simulink model "FIR"  (R2018a)
settings: Solver=VariableStepAuto  StartTime=0.0  StopTime=0.005  RelTol=1e-3
libraries: xbsIndex_r4 x51
settings Model: Creator=57315  LastModifiedBy=57315

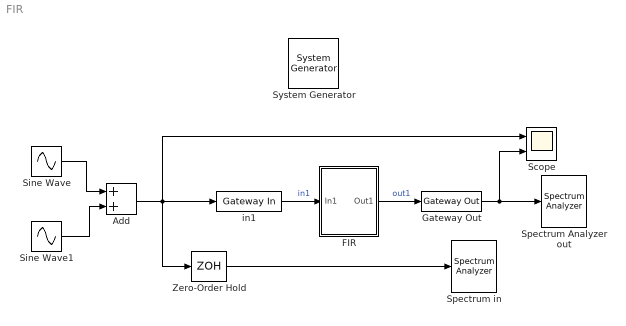
== system FIR ==
  " System Generator" : xbsIndex_r4/ System Generator  Tag=genX  xilinxfamily=kintex7  part=xc7k325t  speed=-3  package=fbg676  synthesis_tool=Vivado  clock_wrapper=Clock Enables  directory=G:/a_max/max_xilinx/max/System_Generator/FIR/FIR3/par  proj_type=Vivado  Synth_file=Vivado Synthesis Defaults  Impl_file=Vivado Implementation Defaults  testbench=on  simulink_period=1/50e6  sysclk_period=20  dcm_input_clock_period=10  incr_netlist=off  trim_vbits=Everywhere in SubSystem  dbl_ovrd=According to Block Masks  core_generation=According to Block Masks  run_coregen=off  deprecated_control=off  eval_field=0  block_type=sysgen
  Add : Sum
  "FIR " : Subsystem
  Gateway Out : xbsIndex_r4/Gateway Out  inherit_from_input=off  hdl_port=on  rows=1  columns=1  UseAsDAC=off  DACChannel='1'  interface=None  automatic_assignment=on  address_offset=hex2dec('00')  intf_name=''  intf_description=''  timing_constraint=None  locs_specified=off  LOCs={}  io_standard={}  block_type=gatewayout
  Scope : Scope  NumInputPorts=2
  Sine Wave : Sin  Frequency=2*pi*1e6  SampleTime=0
  Sine Wave1 : Sin  Frequency=2*pi*9e6  SampleTime=0
  Spectrum Analyzer out : SpectrumAnalyzer
  Spectrum in : SpectrumAnalyzer
  Zero-Order Hold : ZeroOrderHold  SampleTime=1/50e6
  in1 : xbsIndex_r4/Gateway In  gui_display_data_type=Fixed-point  arith_type="Signed  (2's comp)"  n_bits=16  bin_pt=14  preci_type=Single  exp_width=8  frac_width=24  rows=1  columns=1  quantization="Round  (unbiased: +/- Inf)"  overflow=Saturate  period=1/50e6  UseAsADC=off  ADCChannel='1'  interface=None  automatic_assignment=on  address_offset=hex2dec('00')  intf_name=''  intf_description=''  default_value=0  timing_constraint=None  locs_specified=off  LOCs={}  io_standard={}  inherit_from_input=off  hdl_port=on  dbl_ovrd=off  block_type=gatewayin
  wires:
  in1/1 -> "FIR "/1(In1)  "in1"
  Sine Wave/1 -> Add/1
  Sine Wave1/1 -> Add/2
  Add/1 -> Scope/1, Zero-Order Hold/1, in1/1
  Gateway Out/1 -> Scope/2, Spectrum Analyzer out/1
  Zero-Order Hold/1 -> Spectrum in/1
  "FIR "/1(Out1) -> Gateway Out/1  "out1"

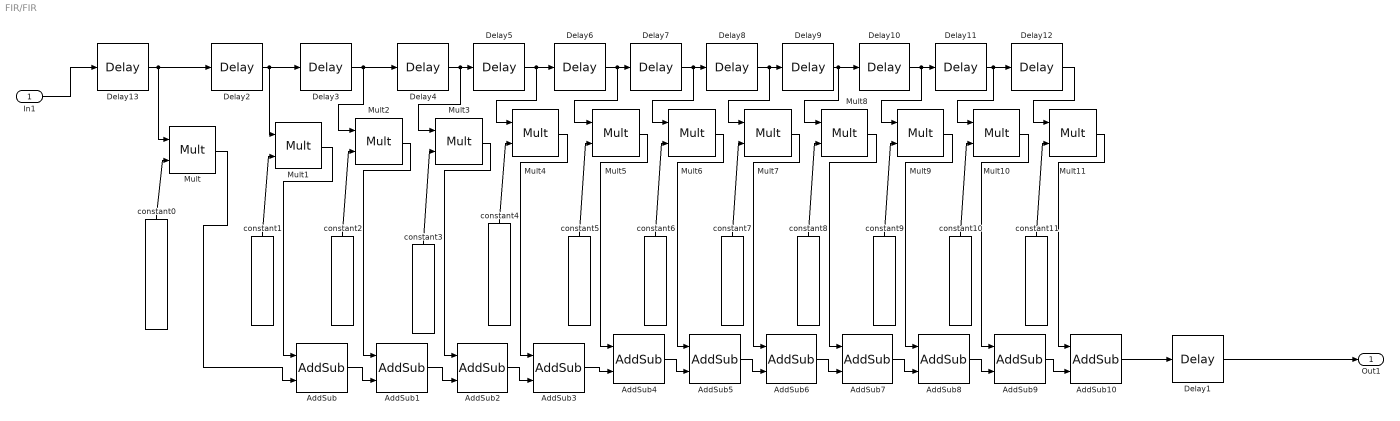
== system FIR/FIR  ==
  In1 : Inport
  AddSub : xbsIndex_r4/AddSub  mode=Addition  use_carryin=off  use_carryout=off  en=off  latency=0  precision=Full  arith_type=Unsigned  n_bits=16  bin_pt=14  quantization=Truncate  overflow=Wrap  use_behavioral_HDL=off  hw_selection=Fabric  pipelined=off  dbl_ovrd=off  block_type=addsub
  AddSub{1..10} (10 alike) : xbsIndex_r4/AddSub  mode=Addition  use_carryin=off  use_carryout=off  en=off  latency=1  precision=Full  arith_type=Unsigned  n_bits=16  bin_pt=14  quantization=Truncate  overflow=Wrap  use_behavioral_HDL=off  hw_selection=Fabric  pipelined=off  dbl_ovrd=off  block_type=addsub
  Delay1 : xbsIndex_r4/Delay  rst=off  infoeditControl=Selection of Reset will increase slice count due to use of real FFs and instead of SRLs  en=off  latency=1  reg_retiming=off  dbl_ovrd=off  block_type=delay
  Delay{2..12} (11 alike) : xbsIndex_r4/Delay  rst=off  infoeditControl=Selection of Reset will increase slice count due to use of real FFs and instead of SRLs  en=off  latency=2  reg_retiming=off  dbl_ovrd=off  block_type=delay
  Delay13 : xbsIndex_r4/Delay  rst=off  infoeditControl=Selection of Reset will increase slice count due to use of real FFs and instead of SRLs  en=off  latency=1  reg_retiming=off  dbl_ovrd=off  block_type=delay
  Mult{,1..11} (12 alike) : xbsIndex_r4/Mult  precision=Full  arith_type="Signed  (2's comp)"  n_bits=16  bin_pt=14  quantization=Truncate  overflow=Wrap  en=off  latency=3  use_behavioral_HDL=off  opt=Speed  use_embedded=on  optimum_pipeline=off  pipeline=on  dbl_ovrd=off  use_rpm=on  placement_style=Triangular  block_type=mult
  constant0 : xbsIndex_r4/Constant  const=1.242e-02  gui_display_data_type=Fixed-point  arith_type=Signed (2's comp)  n_bits=16  bin_pt=14  preci_type=Single  exp_width=8  frac_width=24  explicit_period=off  period=1  equ=P=C  opselect=C  inp2=PCIN>>17  opr=+  inp1=P  carry=CIN  dbl_ovrd=off  block_type=constant
  constant1 : xbsIndex_r4/Constant  const=2.442e-02  gui_display_data_type=Fixed-point  arith_type=Signed (2's comp)  n_bits=16  bin_pt=14  preci_type=Single  exp_width=8  frac_width=24  explicit_period=off  period=1  equ=P=C  opselect=C  inp2=PCIN>>17  opr=+  inp1=P  carry=CIN  dbl_ovrd=off  block_type=constant
  constant10 : xbsIndex_r4/Constant  const=2.442e-02  gui_display_data_type=Fixed-point  arith_type=Signed (2's comp)  n_bits=16  bin_pt=14  preci_type=Single  exp_width=8  frac_width=24  explicit_period=off  period=1  equ=P=C  opselect=C  inp2=PCIN>>17  opr=+  inp1=P  carry=CIN  dbl_ovrd=off  block_type=constant
  constant11 : xbsIndex_r4/Constant  const=1.242e-02  gui_display_data_type=Fixed-point  arith_type=Signed (2's comp)  n_bits=16  bin_pt=14  preci_type=Single  exp_width=8  frac_width=24  explicit_period=off  period=1  equ=P=C  opselect=C  inp2=PCIN>>17  opr=+  inp1=P  carry=CIN  dbl_ovrd=off  block_type=constant
  constant2 : xbsIndex_r4/Constant  const=5.688e-02  gui_display_data_type=Fixed-point  arith_type=Signed (2's comp)  n_bits=16  bin_pt=14  preci_type=Single  exp_width=8  frac_width=24  explicit_period=off  period=1  equ=P=C  opselect=C  inp2=PCIN>>17  opr=+  inp1=P  carry=CIN  dbl_ovrd=off  block_type=constant
  constant3 : xbsIndex_r4/Constant  const=.1003  gui_display_data_type=Fixed-point  arith_type=Signed (2's comp)  n_bits=16  bin_pt=14  preci_type=Single  exp_width=8  frac_width=24  explicit_period=off  period=1  equ=P=C  opselect=C  inp2=PCIN>>17  opr=+  inp1=P  carry=CIN  dbl_ovrd=off  block_type=constant
  constant4 : xbsIndex_r4/Constant  const=0.1408  gui_display_data_type=Fixed-point  arith_type=Signed (2's comp)  n_bits=16  bin_pt=14  preci_type=Single  exp_width=8  frac_width=24  explicit_period=off  period=1  equ=P=C  opselect=C  inp2=PCIN>>17  opr=+  inp1=P  carry=CIN  dbl_ovrd=off  block_type=constant
  constant5 : xbsIndex_r4/Constant  const=.1652  gui_display_data_type=Fixed-point  arith_type=Signed (2's comp)  n_bits=16  bin_pt=14  preci_type=Single  exp_width=8  frac_width=24  explicit_period=off  period=1  equ=P=C  opselect=C  inp2=PCIN>>17  opr=+  inp1=P  carry=CIN  dbl_ovrd=off  block_type=constant
  constant6 : xbsIndex_r4/Constant  const=.1625  gui_display_data_type=Fixed-point  arith_type=Signed (2's comp)  n_bits=16  bin_pt=14  preci_type=Single  exp_width=8  frac_width=24  explicit_period=off  period=1  equ=P=C  opselect=C  inp2=PCIN>>17  opr=+  inp1=P  carry=CIN  dbl_ovrd=off  block_type=constant
  constant7 : xbsIndex_r4/Constant  const=.1408  gui_display_data_type=Fixed-point  arith_type=Signed (2's comp)  n_bits=16  bin_pt=14  preci_type=Single  exp_width=8  frac_width=24  explicit_period=off  period=1  equ=P=C  opselect=C  inp2=PCIN>>17  opr=+  inp1=P  carry=CIN  dbl_ovrd=off  block_type=constant
  constant8 : xbsIndex_r4/Constant  const=.1003  gui_display_data_type=Fixed-point  arith_type=Signed (2's comp)  n_bits=16  bin_pt=14  preci_type=Single  exp_width=8  frac_width=24  explicit_period=off  period=1  equ=P=C  opselect=C  inp2=PCIN>>17  opr=+  inp1=P  carry=CIN  dbl_ovrd=off  block_type=constant
  constant9 : xbsIndex_r4/Constant  const=5.688e-02  gui_display_data_type=Fixed-point  arith_type=Signed (2's comp)  n_bits=16  bin_pt=14  preci_type=Single  exp_width=8  frac_width=24  explicit_period=off  period=1  equ=P=C  opselect=C  inp2=PCIN>>17  opr=+  inp1=P  carry=CIN  dbl_ovrd=off  block_type=constant
  Out1 : Outport
  wires:
  AddSub2/1 -> AddSub3/2
  Mult6/1 -> AddSub5/1
  Delay4/1 -> Delay5/1, Mult3/1
  In1/1 -> Delay13/1
  AddSub/1 -> AddSub1/2
  AddSub3/1 -> AddSub4/2
  constant1/1 -> Mult1/2
  Delay2/1 -> Delay3/1, Mult1/1
  Mult10/1 -> AddSub9/1
  constant6/1 -> Mult6/2
  Mult3/1 -> AddSub2/1
  Mult2/1 -> AddSub1/1
  constant2/1 -> Mult2/2
  Delay13/1 -> Mult/1, Delay2/1
  Mult1/1 -> AddSub/1
  Delay6/1 -> Delay7/1, Mult5/1
  constant3/1 -> Mult3/2
  AddSub9/1 -> AddSub10/2
  Mult11/1 -> AddSub10/1
  Mult/1 -> AddSub/2
  constant9/1 -> Mult9/2
  Delay1/1 -> Out1/1
  constant7/1 -> Mult7/2
  constant0/1 -> Mult/2
  constant8/1 -> Mult8/2
  AddSub6/1 -> AddSub7/2
  AddSub1/1 -> AddSub2/2
  constant4/1 -> Mult4/2
  Delay12/1 -> Mult11/1
  AddSub10/1 -> Delay1/1
  AddSub7/1 -> AddSub8/2
  Delay9/1 -> Mult8/1, Delay10/1
  constant11/1 -> Mult11/2
  Delay8/1 -> Delay9/1, Mult7/1
  Mult5/1 -> AddSub4/1
  Delay11/1 -> Mult10/1, Delay12/1
  Mult7/1 -> AddSub6/1
  constant10/1 -> Mult10/2
  Delay3/1 -> Delay4/1, Mult2/1
  Delay7/1 -> Delay8/1, Mult6/1
  Mult8/1 -> AddSub7/1
  Mult4/1 -> AddSub3/1
  AddSub4/1 -> AddSub5/2
  constant5/1 -> Mult5/2
  AddSub5/1 -> AddSub6/2
  AddSub8/1 -> AddSub9/2
  Mult9/1 -> AddSub8/1
  Delay5/1 -> Delay6/1, Mult4/1
  Delay10/1 -> Delay11/1, Mult9/1
